simulink model "sim_tase_2025_pos_ctrl"  (R2020a)
settings: Solver=ode4  StartTime=0.0  StopTime=30.0  FixedStep=0.01  RelTol=1e-3
values from neighbouring files (symbols this model uses):
  alfa_theta_obs = 100    [init_tase_2025_pos_ctrl.m]
  Aps = -diag([5, 5, 5])    [init_tase_2025_pos_ctrl.m]
  delta_p_i_0 = zeros(3, NF)    [init_tase_2025_pos_ctrl.m]
  delta_v_i_0 = zeros(3, NF)    [init_tase_2025_pos_ctrl.m]
  dp_aa_t = 0.2 * ones(3, 5) + ( 1.0 - 0.2 ) * rand(3, 5)    [init_tase_2025_pos_ctrl.m]
  dp_ff_t = [ 0.4 * ones(1, 5) + ( 1.0 - 0.4 ) * rand(1, 5);                      0.4 * ones(1, 5) + ( 1.0 - 0.4 ) * rand(1, 5);                      0.2 * ones(1, 5) + ( 0.6 - 0.2 ) * rand(1, 5) ]    [init_tase_2025_pos_ctrl.m]
  dp_phi_t = ( - pi / 2 ) * ones(3, 5) + ( pi / 2 - ( - pi / 2 ) ) * rand(3, 5)    [init_tase_2025_pos_ctrl.m]
  etai_0 = zeros(3,5)    [init_tase_2025_pos_ctrl.m]
  k_rho_1 = 10    [init_tase_2025_pos_ctrl.m]
  k_rho_2 = 10    [init_tase_2025_pos_ctrl.m]
  kai_1_t = 0.02    [init_tase_2025_pos_ctrl.m]
  kai_3_t = 0.1    [init_tase_2025_pos_ctrl.m]
  kp = 20    [init_tase_2025_pos_ctrl.m]
  ksii_0 = zeros(3,5)    [init_tase_2025_pos_ctrl.m]
  kv = 20    [init_tase_2025_pos_ctrl.m]
  l1v = diag([20; 20; 20])    [init_tase_2025_pos_ctrl.m]
  l2v = diag([30; 30; 30])    [init_tase_2025_pos_ctrl.m]
  mass_i = zeros(1,NF)    [init_tase_2025_pos_ctrl.m]
  Mii = diag([1;0;0;0;1])    [init_tase_2025_pos_ctrl.m]
  Phi_inv = inv( Aps ) * ( exp( Aps * tTs ) - eye(3) )    [init_tase_2025_pos_ctrl.m]
  pos0 = zeros(3, 1)    [init_tase_2025_pos_ctrl.m]
  PZ0 = P0(3)    [init_tase_2025_pos_ctrl.m]
  PZ1 = 10    [init_tase_2025_pos_ctrl.m]
  Qci_init = repmat([1;0;0;0],1,NF)    [init_tase_2025_pos_ctrl.m]
  R0 = 4    [init_tase_2025_pos_ctrl.m]
  R1 = 8    [init_tase_2025_pos_ctrl.m]
  Rx2 = 10    [init_tase_2025_pos_ctrl.m]
  Ry2 = 6    [init_tase_2025_pos_ctrl.m]
  Rz2 = 4    [init_tase_2025_pos_ctrl.m]
  T0 = 0    [init_tase_2025_pos_ctrl.m]
  T1 = tseq1    (= 10)    [init_tase_2025_pos_ctrl.m]
  T12 = tseq1 + tseq12    (= 20)    [init_tase_2025_pos_ctrl.m]
  T2 = tseq1 + tseq12 + tseq2    (= 30)    [init_tase_2025_pos_ctrl.m]
  theta0 = ( 2 / 5 ) * pi    (= 1.25663706144)    [init_tase_2025_pos_ctrl.m]
  theta_1 = 0    [init_tase_2025_pos_ctrl.m]
  theta_2 = 1    [init_tase_2025_pos_ctrl.m]
  TTb = 2    [init_tase_2025_pos_ctrl.m]
  tTs = 0.1    [init_tase_2025_pos_ctrl.m]
  vel0 = zeros(3, 1)    [init_tase_2025_pos_ctrl.m]
  Wij = [0,0,1,0,0;              0,0,1,1,0;              1,0,0,0,1;              0,1,1,0,0;              0,0,1,0,0]    [init_tase_2025_pos_ctrl.m]
  wp = 10    [init_tase_2025_pos_ctrl.m]
  X1 = 8    [init_tase_2025_pos_ctrl.m]
  X2 = 2    [init_tase_2025_pos_ctrl.m]
  X3 = 3    [init_tase_2025_pos_ctrl.m]
  Y1 = 10    [init_tase_2025_pos_ctrl.m]
  Y2 = 2    [init_tase_2025_pos_ctrl.m]
  Y3 = 4    [init_tase_2025_pos_ctrl.m]
  Z1 = 4    [init_tase_2025_pos_ctrl.m]
  Z2 = -6    [init_tase_2025_pos_ctrl.m]
  Z3 = 2    [init_tase_2025_pos_ctrl.m]
undefined symbols (not defined in the file or in its folder): cal_frac_squ, p_gamma1_pos, p_gamma1_vel, p_gamma2_pos, p_gamma2_vel, p_gamma_diff_1, p_gamma_diff_2_2, q_gamma1_pos, q_gamma1_vel, q_gamma2_pos, q_gamma2_vel, q_gamma_diff_1, q_gamma_diff_2_2
(part 4 of 4)

== matlab function sim_tase_2025_pos_ctrl/combine sig_ksi_diff_tilt_gamma_2_2 ==
  data: sig_ksi_diff_tilt_gamma_2_2_node_1 input; sig_ksi_diff_tilt_gamma_2_2_vec output; sig_ksi_diff_tilt_gamma_2_2_node_2 input; sig_ksi_diff_tilt_gamma_2_2_node_3 input; sig_ksi_diff_tilt_gamma_2_2_node_4 input; sig_ksi_diff_tilt_gamma_2_2_node_5 input
function sig_ksi_diff_tilt_gamma_2_2_vec = fcn(sig_ksi_diff_tilt_gamma_2_2_node_1, sig_ksi_diff_tilt_gamma_2_2_node_2, ...
                                                                                        sig_ksi_diff_tilt_gamma_2_2_node_3, sig_ksi_diff_tilt_gamma_2_2_node_4, ...
                                                                                        sig_ksi_diff_tilt_gamma_2_2_node_5)
%%%% 合并绝对值幂次项
sig_ksi_diff_tilt_gamma_2_2_vec = zeros(3,5);
sig_ksi_diff_tilt_gamma_2_2_vec(:,1) = sig_ksi_diff_tilt_gamma_2_2_node_1(:);
sig_ksi_diff_tilt_gamma_2_2_vec(:,2) = sig_ksi_diff_tilt_gamma_2_2_node_2(:);
sig_ksi_diff_tilt_gamma_2_2_vec(:,3) = sig_ksi_diff_tilt_gamma_2_2_node_3(:);
sig_ksi_diff_tilt_gamma_2_2_vec(:,4) = sig_ksi_diff_tilt_gamma_2_2_node_4(:);
sig_ksi_diff_tilt_gamma_2_2_vec(:,5) = sig_ksi_diff_tilt_gamma_2_2_node_5(:);

== matlab function sim_tase_2025_pos_ctrl/cal vel_diff_hat agent 2 ==
  data: k_rho_1 input; k_rho_2 input; TTb input; theta_1 input; theta_2 input; tsim input; ksi_diff_tilt_vec input; d_vel_diff_hat_2 output; sig_ksi_diff_tilt_gamma_1_vec input
function d_vel_diff_hat_2 = fcn(k_rho_1, k_rho_2, TTb, theta_1, theta_2, tsim, ksi_diff_tilt_vec, sig_ksi_diff_tilt_gamma_1_vec)
%%%% 计算高阶滑模微分器的速度估计
iiuav = 2;
if tsim < TTb
    theta = theta_1;
else
    theta = theta_2;
end
d_vel_diff_hat_2 = -theta * k_rho_1 * sign( ksi_diff_tilt_vec(:,iiuav) ) ...
                                    - ( 1 - theta ) * k_rho_2 * sig_ksi_diff_tilt_gamma_1_vec(:,iiuav);
